simulink model "Controllo_assey_4gdl_discretizzato"  (R2021a)
settings: Solver=VariableStepAuto  StartTime=0.0  StopTime=2  RelTol=1e-3
values from neighbouring files (symbols this model uses):
  my = config_dc(pary)    [mainy.m]
  pary = parametriy ()    [mainy.m]
undefined symbols (not defined in the file or in its folder): accelerazioniy, Evaluate_Trajectory
libraries: cstblocks x4, simulink x2
settings Model: Creator=stefa  LastModifiedBy=stefa

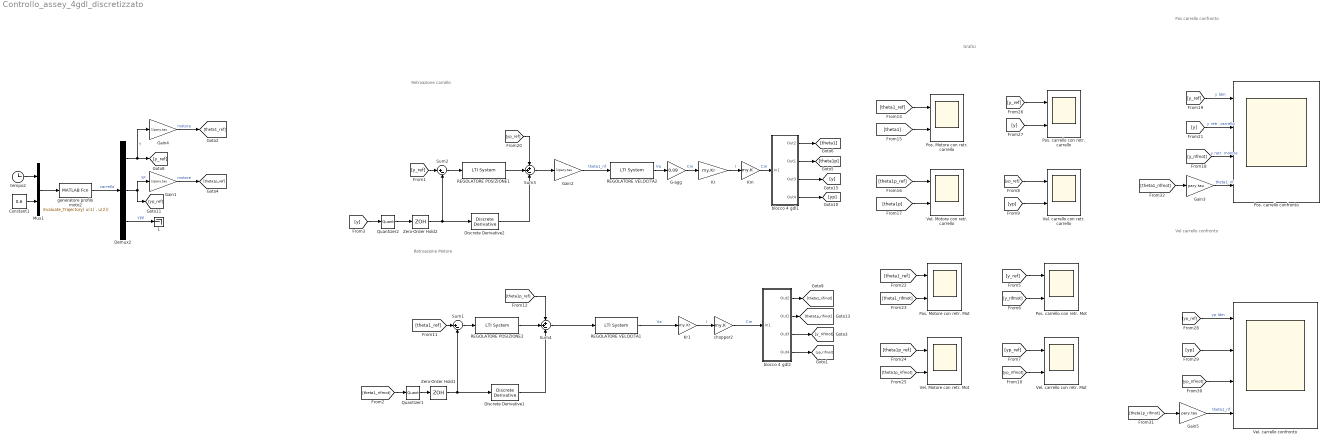
== system Controllo_assey_4gdl_discretizzato ==
  note: Grafici
  note: Retroazione carrello
  note: Retroazione Motore
  note: Pos carrello confronto
  note: Vel carrello confronto
  " 1" : Terminator
  Constant1 : Constant  Value=0.6
  Demux2 : Demux  Outputs=3
  Discrete Derivative1 : simulink/Discrete/Discrete Derivative  gainval=1.0  ICPrevScaledInput=0.0  OutMin=[]  OutMax=[]  OutDataType=fixdt(1, 16)  OutScaling=2^-10  DoSatur=off
  Discrete Derivative2 : simulink/Discrete/Discrete Derivative  gainval=1.0  ICPrevScaledInput=0.0  OutMin=[]  OutMax=[]  OutDataType=fixdt(1, 16)  OutScaling=2^-10  DoSatur=off
  G-agg : Gain  Gain=0.09
  Gain1 : Gain  Gain=1/pary.tau
  Gain2 : Gain  Gain=1/pary.tau
  Gain3 : Gain  Gain=pary.tau
  Gain4 : Gain  Gain=1/pary.tau
  Gain5 : Gain  Gain=pary.tau
  Km : Gain  Gain=my.K
  Kr : Gain  Gain=my.Kr
  Kr1 : Gain  Gain=my.Kr
  Mux1 : Mux  Inputs=2
  Pos. Motore con retr. Mot : Scope  NumInputPorts=2
  Pos. Motore con retr. carrello : Scope  NumInputPorts=2
  Pos. carrello con retr. Mot : Scope  NumInputPorts=2
  Pos. carrello con retr. carrello : Scope  NumInputPorts=2
  Pos. carrello confronto : Scope  NumInputPorts=4
  Quantizer1 : Quantizer  QuantizationInterval=10/4096
  Quantizer2 : Quantizer  QuantizationInterval=10/4096
  REGOLATORE POSIZIONE1 : cstblocks/LTI System  sys=ap.H_P  IC=[]
  REGOLATORE POSIZIONE2 : cstblocks/LTI System  sys=ap.H_P  IC=[]
  REGOLATORE VELOCITA1 : cstblocks/LTI System  sys=av.PI_V  IC=[]
  REGOLATORE VELOCITA2 : cstblocks/LTI System  sys=av.PI_V  IC=[]
  Sum1 : Sum  Inputs=|+-
  Sum2 : Sum  Inputs=|+-
  Sum3 : Sum  Inputs=++-
  Sum4 : Sum  Inputs=++-
  Vel. Motore con retr. Mot : Scope  NumInputPorts=2
  Vel. Motore con retr. carrello : Scope  NumInputPorts=2
  Vel. carrello con retr. Mot : Scope  NumInputPorts=2
  Vel. carrello con retr. carrello : Scope  NumInputPorts=2
  Vel. carrello confronto : Scope  NumInputPorts=4
  Zero-Order Hold1 : ZeroOrderHold  SampleTime=0.001
  Zero-Order Hold2 : ZeroOrderHold  SampleTime=0.001
  blocco 4 gdl1 : Subsystem
  blocco 4 gdl2 : Subsystem
  chopper2 : Gain  Gain=my.K
  generatore profilo moto2 : MATLABFcn  MATLABFcn=Evaluate_Trajectory( u(1) , u(2))  OutputDimensions=3
  tempo2 : Clock
  wires:
  Gain5/1 -> Vel. carrello confronto/4  "theta1_rif"
  [y_ref] -> Pos. carrello confronto/1  "y ldm"
  [yp] -> Vel. carrello confronto/2
  [y] -> Pos. carrello confronto/2  "y retr. carrello"
  [y] -> Pos. carrello con retr. carrello/2
  [yp_rifmot] -> Vel. carrello confronto/3
  blocco 4 gdl2/4(Out4) -> [yp_rifmot]
  [theta1_rifmot] -> Pos. Motore con retr. Mot/2
  [theta1_ref] -> Pos. Motore con retr. carrello/1
  [theta1p_ref] -> Vel. Motore con retr. carrello/1
  [theta1] -> Pos. Motore con retr. carrello/2
  [theta1_ref] -> Sum1/1
  [y_rifmot] -> Pos. carrello confronto/3  "y retr. motore"
  blocco 4 gdl2/1(Out2) -> [theta1_rifmot]
  Gain4/1 -> [theta1_ref]  "motore"
  Discrete Derivative1/1 -> Sum4/3
  [y_ref] -> Pos. carrello con retr. Mot/1
  Km/1 -> blocco 4 gdl1/1(In1)  "Cm"
  [theta1p_rifmot] -> Vel. Motore con retr. Mot/2
  Gain1/1 -> [theta1p_ref]  "motore"
  chopper2/1 -> blocco 4 gdl2/1(In1)  "Cm"
  Gain2/1 -> REGOLATORE VELOCITA2/1  "theta1_rif"
  [theta1p_ref] -> Sum4/1
  [theta1_ref] -> Pos. Motore con retr. Mot/1
  Sum3/1 -> Gain2/1
  Discrete Derivative2/1 -> Sum3/3
  REGOLATORE VELOCITA1/1 -> Kr1/1  "Va"
  [yp_ref] -> Vel. carrello con retr. carrello/1
  Sum1/1 -> REGOLATORE POSIZIONE2/1
  [y_ref] -> Sum2/1
  REGOLATORE POSIZIONE2/1 -> Sum4/2
  blocco 4 gdl1/1(Out2) -> [theta1]
  Demux2/1 -> [y_ref], Gain4/1  "Y"
  blocco 4 gdl2/3(Out3) -> [y_rifmot]
  [yp_ref] -> Sum3/1
  [yp_ref] -> Vel. carrello confronto/1  "yp ldm"
  Demux2/2 -> Gain1/1, [yp_ref]  "YP"
  [theta1p_ref] -> Vel. Motore con retr. Mot/1
  [y_ref] -> Pos. carrello con retr. carrello/1
  Sum2/1 -> REGOLATORE POSIZIONE1/1
  tempo2/1 -> Mux1/1
  [yp_ref] -> Vel. carrello con retr. Mot/1
  Mux1/1 -> generatore profilo moto2/1
  [theta1p] -> Vel. Motore con retr. carrello/2
  Demux2/3 -> " 1"/1  "YPP"
  [yp_rifmot] -> Vel. carrello con retr. Mot/2
  blocco 4 gdl1/4(Out4) -> [yp]
  [yp] -> Vel. carrello con retr. carrello/2
  generatore profilo moto2/1 -> Demux2/1  "carrello"
  blocco 4 gdl2/2(Out1) -> [theta1p_rifmot]
  Constant1/1 -> Mux1/2
  REGOLATORE POSIZIONE1/1 -> Sum3/2
  Kr/1 -> Km/1  "I"
  Sum4/1 -> REGOLATORE VELOCITA1/1
  Gain3/1 -> Pos. carrello confronto/4  "theta1_rif"
  [theta1p_rifmot] -> Gain5/1
  Zero-Order Hold1/1 -> Discrete Derivative1/1, Sum1/2
  [theta1_rifmot] -> Gain3/1
  blocco 4 gdl1/2(Out1) -> [theta1p]
  Kr1/1 -> chopper2/1  "I"
  blocco 4 gdl1/3(Out3) -> [y]
  [y_rifmot] -> Pos. carrello con retr. Mot/2
  [y] -> Quantizer2/1
  Quantizer2/1 -> Zero-Order Hold2/1
  Zero-Order Hold2/1 -> Discrete Derivative2/1, Sum2/2
  Quantizer1/1 -> Zero-Order Hold1/1
  [theta1_rifmot] -> Quantizer1/1
  REGOLATORE VELOCITA2/1 -> G-agg/1  "Va"
  G-agg/1 -> Kr/1  "Cm"

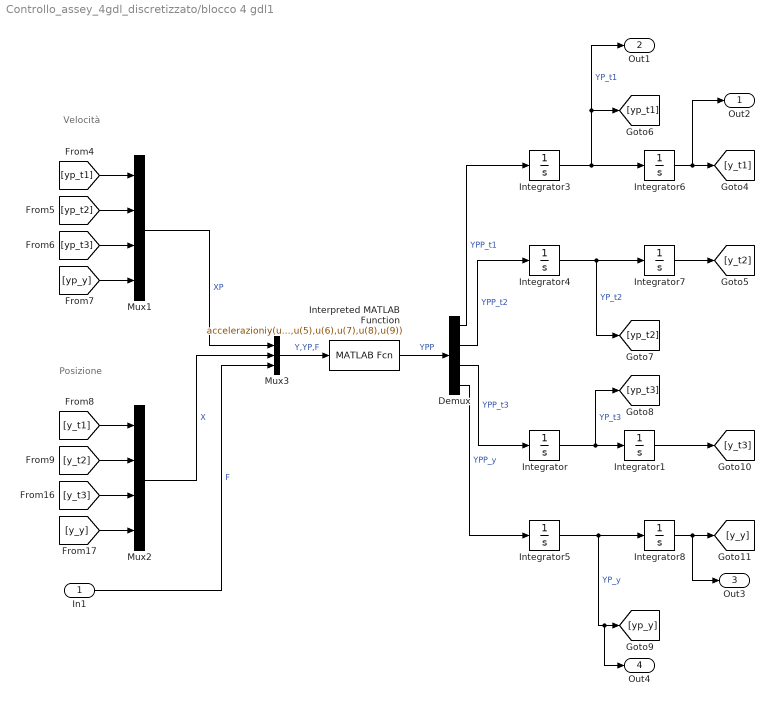
== system Controllo_assey_4gdl_discretizzato/blocco 4 gdl1 ==
  note: Posizione
  note: Velocità
  In1 : Inport
  Demux : Demux
  Integrator{,1,3..7} (7 alike) : Integrator
  Integrator8 : Integrator  InitialCondition=0.0005
  Interpreted MATLAB Function : MATLABFcn  MATLABFcn=accelerazioniy(u(1),u(2),u(3),u(4),u(5),u(6),u(7),u(8),u(9))  OutputDimensions=4
  Mux1 : Mux
  Mux2 : Mux
  Mux3 : Mux  Inputs=3
  Out2 : Outport
  Out1 : Outport  Port=2
  Out3 : Outport  Port=3
  Out4 : Outport  Port=4
  wires:
  Integrator/1 -> Integrator1/1, [yp_t3]  "YP_t3"
  Mux1/1 -> Mux3/1  "XP"
  [y_t3] -> Mux2/3
  Mux3/1 -> Interpreted MATLAB Function/1  "Y,YP,F"
  [y_t2] -> Mux2/2
  Integrator7/1 -> [y_t2]
  Demux/3 -> Integrator/1  "YPP_t3"
  [yp_y] -> Mux1/4
  [y_y] -> Mux2/4
  Demux/1 -> Integrator3/1  "YPP_t1"
  [yp_t2] -> Mux1/2
  Mux2/1 -> Mux3/2  "X"
  Interpreted MATLAB Function/1 -> Demux/1  "YPP"
  Integrator8/1 -> Out3/1, [y_y]
  Integrator4/1 -> [yp_t2], Integrator7/1  "YP_t2"
  Integrator3/1 -> Out1/1, [yp_t1], Integrator6/1  "YP_t1"
  In1/1 -> Mux3/3  "F"
  Demux/2 -> Integrator4/1  "YPP_t2"
  Integrator5/1 -> Out4/1, [yp_y], Integrator8/1  "YP_y"
  Integrator6/1 -> Out2/1, [y_t1]
  [yp_t3] -> Mux1/3
  Demux/4 -> Integrator5/1  "YPP_y"
  Integrator1/1 -> [y_t3]
  [yp_t1] -> Mux1/1
  [y_t1] -> Mux2/1

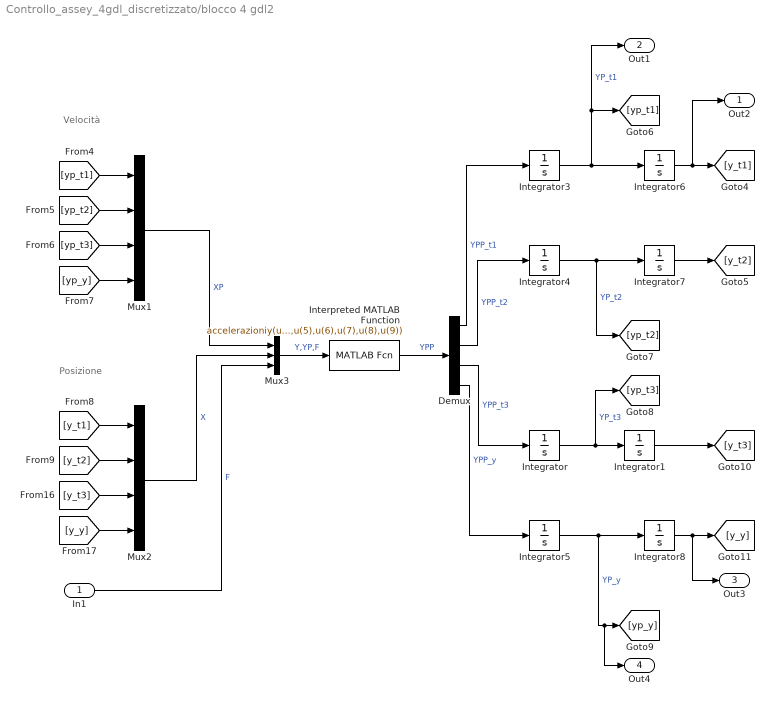
== system Controllo_assey_4gdl_discretizzato/blocco 4 gdl2 ==
  note: Posizione
  note: Velocità
  In1 : Inport
  Demux : Demux
  Integrator{,1,3..7} (7 alike) : Integrator
  Integrator8 : Integrator  InitialCondition=0.0005
  Interpreted MATLAB Function : MATLABFcn  MATLABFcn=accelerazioniy(u(1),u(2),u(3),u(4),u(5),u(6),u(7),u(8),u(9))  OutputDimensions=4
  Mux1 : Mux
  Mux2 : Mux
  Mux3 : Mux  Inputs=3
  Out2 : Outport
  Out1 : Outport  Port=2
  Out3 : Outport  Port=3
  Out4 : Outport  Port=4
  wires:
  Integrator/1 -> Integrator1/1, [yp_t3]  "YP_t3"
  Mux1/1 -> Mux3/1  "XP"
  [y_t3] -> Mux2/3
  Mux3/1 -> Interpreted MATLAB Function/1  "Y,YP,F"
  [y_t2] -> Mux2/2
  Integrator7/1 -> [y_t2]
  Demux/3 -> Integrator/1  "YPP_t3"
  [yp_y] -> Mux1/4
  [y_y] -> Mux2/4
  Demux/1 -> Integrator3/1  "YPP_t1"
  [yp_t2] -> Mux1/2
  Mux2/1 -> Mux3/2  "X"
  Interpreted MATLAB Function/1 -> Demux/1  "YPP"
  Integrator8/1 -> Out3/1, [y_y]
  Integrator4/1 -> [yp_t2], Integrator7/1  "YP_t2"
  Integrator3/1 -> Out1/1, [yp_t1], Integrator6/1  "YP_t1"
  In1/1 -> Mux3/3  "F"
  Demux/2 -> Integrator4/1  "YPP_t2"
  Integrator5/1 -> Out4/1, [yp_y], Integrator8/1  "YP_y"
  Integrator6/1 -> Out2/1, [y_t1]
  [yp_t3] -> Mux1/3
  Demux/4 -> Integrator5/1  "YPP_y"
  Integrator1/1 -> [y_t3]
  [yp_t1] -> Mux1/1
  [y_t1] -> Mux2/1
